simulink model "without_sesnor_feedback"  (R2015a)
settings: Solver=ode45  StartTime=0.0  StopTime=10.0  RelTol=1e-3
libraries: simulink x1
settings Model: Creator=Manoj  LastModifiedBy=Manoj

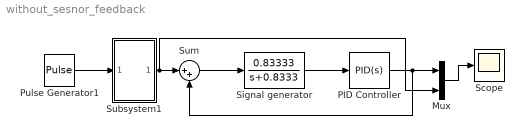
== system without_sesnor_feedback ==
  Mux : Mux  Inputs=2
  PID Controller : simulink/Continuous/PID Controller  Controller=PID  TimeDomain=Continuous-time  SampleTime=-1  IntegratorMethod=Forward Euler  FilterMethod=Forward Euler  Form=Parallel  UseFilter=on  ControllerParametersSource=internal  P=-0.334662045690388  I=-0.742195004649282  D=0  N=100  InitialConditionSource=internal  InitialConditionForIntegrator=0  InitialConditionForFilter=0  ExternalReset=none  LimitOutput=off  UpperSaturationLimit=inf  LowerSaturationLimit=-inf  LinearizeAsGain=on  AntiWindupMode=none  Kb=1  TrackingMode=off  Kt=1  PParamMin=[]  PParamMax=[]  IParamMin=[]  IParamMax=[]  DParamMin=[]  DParamMax=[]  NParamMin=[]  NParamMax=[]  KbParamMin=[]  KbParamMax=[]  KtParamMin=[]  KtParamMax=[]  POutMin=[]  POutMax=[]  IOutMin=[]  IOutMax=[]  DOutMin=[]  DOutMax=[]  NOutMin=[]  NOutMax=[]  KbOutMin=[]  KbOutMax=[]  KtOutMin=[]  KtOutMax=[]  IntegratorOutMin=[]  IntegratorOutMax=[]  FilterOutMin=[]  FilterOutMax=[]  SumOutMin=[]  SumOutMax=[]  SumI1OutMin=[]  SumI1OutMax=[]  SumI2OutMin=[]  SumI2OutMax=[]  SumI3OutMin=[]  SumI3OutMax=[]  SumDOutMin=[]  SumDOutMax=[]  SaturationOutMin=[]  SaturationOutMax=[]  IntegratorContinuousStateAttributes=''  IntegratorStateMustResolveToSignalObject=off  IntegratorRTWStateStorageClass=Auto  FilterContinuousStateAttributes=''  FilterStateMustResolveToSignalObject=off  FilterRTWStateStorageClass=Auto  DifferentiatorICPrevScaledInput=0  DifferentiatorOutMin=[]  DifferentiatorOutMax=[]
  Pulse Generator1 : DiscretePulseGenerator  PulseType=Time based  Period=4  PhaseDelay=0-1
  Scope : Scope
      settings: TimeRange=10  YMin=-0.004  YMax=0.008
  Signal generator : TransferFcn  Numerator=[0.83333]  Denominator=[1 0.8333]
  Subsystem1 : Subsystem
  Sum : Sum  Inputs=|++
  wires:
  Subsystem1/1(Out1) -> Mux/2, Sum/1
  Signal generator/1 -> PID Controller/1
  PID Controller/1 -> Mux/1, Sum/2
  Pulse Generator1/1 -> Subsystem1/1(In1)
  Sum/1 -> Signal generator/1
  Mux/1 -> Scope/1

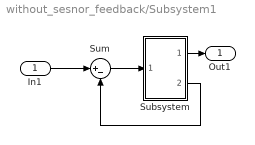
== system without_sesnor_feedback/Subsystem1 ==
  In1 : Inport
  Subsystem : Subsystem
  Sum : Sum  Inputs=|+-
  Out1 : Outport
  wires:
  In1/1 -> Sum/1
  Subsystem/1(Out1) -> Out1/1
  Subsystem/2(Out2) -> Sum/2
  Sum/1 -> Subsystem/1(In1)

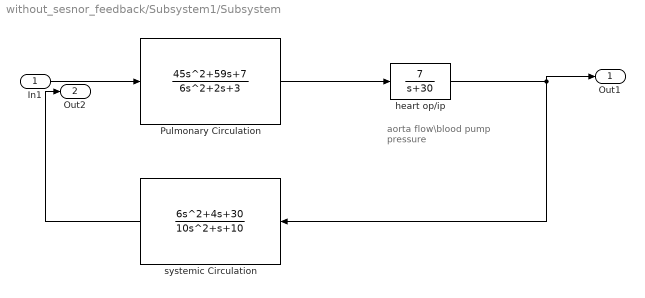
== system without_sesnor_feedback/Subsystem1/Subsystem ==
  note: aorta flow\blood pump pressure
  In1 : Inport
  Pulmonary Circulation : TransferFcn  Numerator=[45 59 7]  Denominator=[6 2 3]
  heart op/ip : TransferFcn  Numerator=[7]  Denominator=[1 30]
  systemic Circulation : TransferFcn  Numerator=[6 4 30]  Denominator=[10 1 10]
  Out1 : Outport
  Out2 : Outport  Port=2
  wires:
  In1/1 -> Pulmonary Circulation/1
  heart op/ip/1 -> systemic Circulation/1, Out1/1
  systemic Circulation/1 -> Out2/1
  Pulmonary Circulation/1 -> heart op/ip/1
